simulink model "demo_integer2Bytes"  (R2020b)
settings: Solver=VariableStepAuto  StartTime=0.0  StopTime=10.0  RelTol=1e-3
libraries: simulink x1
settings Model: Creator=yinti  LastModifiedBy=yinti

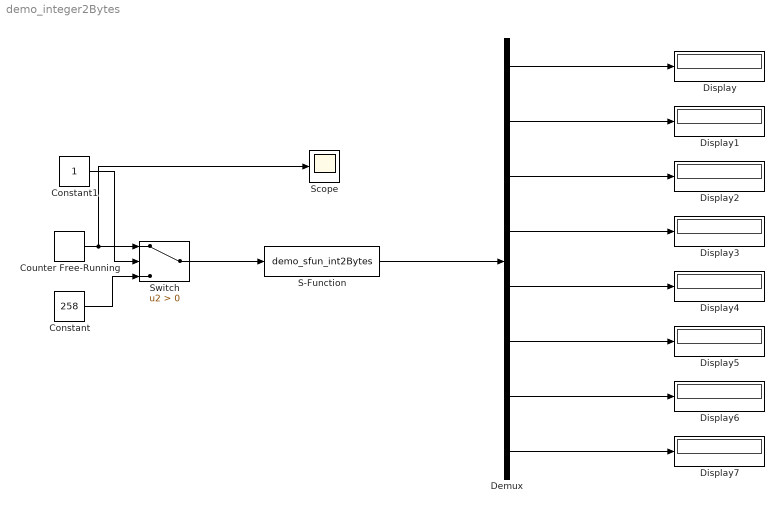
== system demo_integer2Bytes ==
  Constant : Constant  Value=258
  Constant1 : Constant
  Counter Free-Running : simulink/Sources/Counter Free-Running  NumBits=128  tsamp=-1
  Demux : Demux  Outputs=8
  Display{,1..7} (8 alike) : Display
  S-Function : S-Function  FunctionName=demo_sfun_int2Bytes  SFunctionDeploymentMode=off  EnableBusSupport=off
  Scope : Scope
  Switch : Switch  Criteria=u2 > Threshold
  wires:
  Counter Free-Running/1 -> Scope/1, Switch/1
  Constant/1 -> Switch/3
  Constant1/1 -> Switch/2
  Switch/1 -> S-Function/1
  S-Function/1 -> Demux/1
  Demux/2 -> Display1/1
  Demux/3 -> Display2/1
  Demux/4 -> Display3/1
  Demux/5 -> Display4/1
  Demux/6 -> Display5/1
  Demux/7 -> Display6/1
  Demux/8 -> Display7/1
  Demux/1 -> Display/1
